simulink model "LinMotAct_total"  (R2019b)
settings: Solver=FixedStepAuto  StartTime=0.0  StopTime=inf  FixedStep=0.001  RelTol=1e-3  EnableMultiTasking=on
PostLoadFcn:
  | if any(exist('dsrtsu_mdlpostloadfcn', 'file') ~= 0), dsrtsu_mdlpostloadfcn('Execute', bdroot); end
values from neighbouring files (symbols this model uses):
  Ts_Outer = 0.1    [Working_model_LastVersion24_June.m]    (also in model_and_controller.m)
undefined symbols (not defined in the file or in its folder): denc_mi, denco13_dis_des, denF, numc_mi, numco13_dis_des, numF
libraries: rti3002t2lib x6, simulink x4, rtilibm x3, rti4201serlib x3
(part 2 of 2)

== matlab function LinMotAct_total/Actuator/MATLAB Function1 ==
  data: alpha input; beta input; psi input; P_A_ref output; P_B_ref output; P_C_ref output; L_in1 output; L_in2 output; L_in3 output
function [P_A_ref,P_B_ref,P_C_ref,L_in1,L_in2,L_in3] = myfunc(alpha,beta,psi)

%% Rotation matrices

%    Z rotation with angle  psi
RotZ  = [cos(psi) -sin(psi) 0;
         sin(psi)  cos(psi) 0;
          0          0      1]
      
%    Y rotation with angle beta+
RotY  = [cos(beta)       0         sin(beta);
             0           1             0    ;
         -sin(beta)      0        cos(beta)]
    
%    X rotation with angle alpha
RotX  = [1            0                 0    ;
         0        cos(alpha)      -sin(alpha);
         0        sin(alpha)       cos(alpha)]
Rot_BtoP = RotZ*RotY*RotX

%% Specification of the base plate and plate

%Location of motors on the base plate 
r_base = 0.17;               %radii of the base plate (m)
B1     = [r_base; 0; 0]      %position of motor wrt base plate origin
B2     = [-0.5*r_base; (sqrt(3)/2)*r_base; 0]  %120degrees wrt the position of first motor and base plate origin
B3     = [-0.5*r_base; -(sqrt(3)/2)*r_base; 0] %240 degrees wrt first motor and base plate origin

%Location of joints on the plate 
r_plate = 0.17;               %radii of the plate (m)
P1     = [r_plate; 0; 0]      %position of motor wrt base plate origin
P2     = [-0.5*r_plate; (sqrt(3)/2)*r_plate; 0]  %120degrees wrt the position of first motor and base plate origin
P3     = [-0.5*r_plate; -(sqrt(3)/2)*r_plate; 0] %240 degrees wrt first motor and base plate origin

% distance from base plate origin(OXYZ) to plate origin(oxyz)
T = [0; 0; 0.322]                     %30 cm height from (OXYZ) to (oxyz)

%% 
L_in1 = T + (Rot_BtoP*P1)-B1       %change of position of lin motor 1
P_A_ref = sqrt(L_in1(1,1)^2+L_in1(2,1)^2+L_in1(3,1)^2)   %length of L_in1 for passing to motor tf

L_in2 = T + (Rot_BtoP*P2)-B2
P_B_ref = sqrt(L_in2(1,1)^2+L_in2(2,1)^2+L_in2(3,1)^2)

L_in3 = T + (Rot_BtoP*P3)-B3 
P_C_ref = sqrt(L_in3(1,1)^2+L_in3(2,1)^2+L_in3(3,1)^2)
end
